simulink model "motor"  (R2016a)
settings: Solver=VariableStepAuto  StartTime=0.0  StopTime=10.0  RelTol=1e-3
values from neighbouring files (symbols this model uses):
  k = 180    [postavljanje_konstanti.m]
  ki = 0.03    [postavljanje_konstanti.m]
  kp = 0.01    [postavljanje_konstanti.m]
  r_max = 100    [postavljanje_konstanti.m]
  T = 1.2    [postavljanje_konstanti.m]
settings Model: Creator=Vukan  LastModifiedBy=Vukan

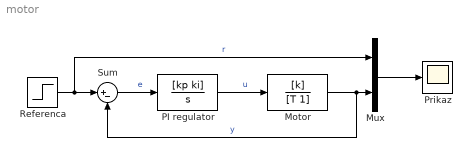
== system motor ==
  Motor : TransferFcn  Numerator=[k]  Denominator=[T 1]
  Mux : Mux  Inputs=2
  PI regulator : TransferFcn  Numerator=[kp ki]  Denominator=[1 0]
  Prikaz : Scope
  Referenca : Step  Time=0  After=r_max  SampleTime=0
  Sum : Sum  Inputs=|+-
  wires:
  Referenca/1 -> Mux/1, Sum/1  "r"
  Sum/1 -> PI regulator/1  "e"
  PI regulator/1 -> Motor/1  "u"
  Mux/1 -> Prikaz/1
  Motor/1 -> Sum/2, Mux/2  "y"
